simulink model "torque_control_model_2_3_2019"  (R2017b)
settings: Solver=VariableStepAuto  StartTime=0.0  StopTime=10  RelTol=1e-3
InitFcn:
  | BLDC_motor_constants_2
values from neighbouring files (symbols this model uses):
  A = [-terminal_resistance/terminal_inductance, 0, 0 ... (first row only)    [BLDC_motor_constants_2.m]    (also in forward_dynamics.m = pinv(Z) * V; inverse_dynamics.m = -pinv(Z) * v)
  B = [2/(3 * terminal_inductance), 1/(3 * terminal_inductance), 0 ... (first row only)    [BLDC_motor_constants_2.m]    (also in forward_dynamics.m = pinv(Z)/gear_ratio)
  C = [1, 0, 0 ... (first row only)    [BLDC_motor_constants_2.m]
  pole_pairs = 8    [BLDC_motor_constants_2.m]
  speed_constant = 259    [BLDC_motor_constants_2.m]
  terminal_resistance = 0.608    [BLDC_motor_constants_2.m]
  torque_constant = 36.9    [BLDC_motor_constants_2.m]
libraries: simulink x2
settings Model: Creator=Zach  LastModifiedBy=Zach

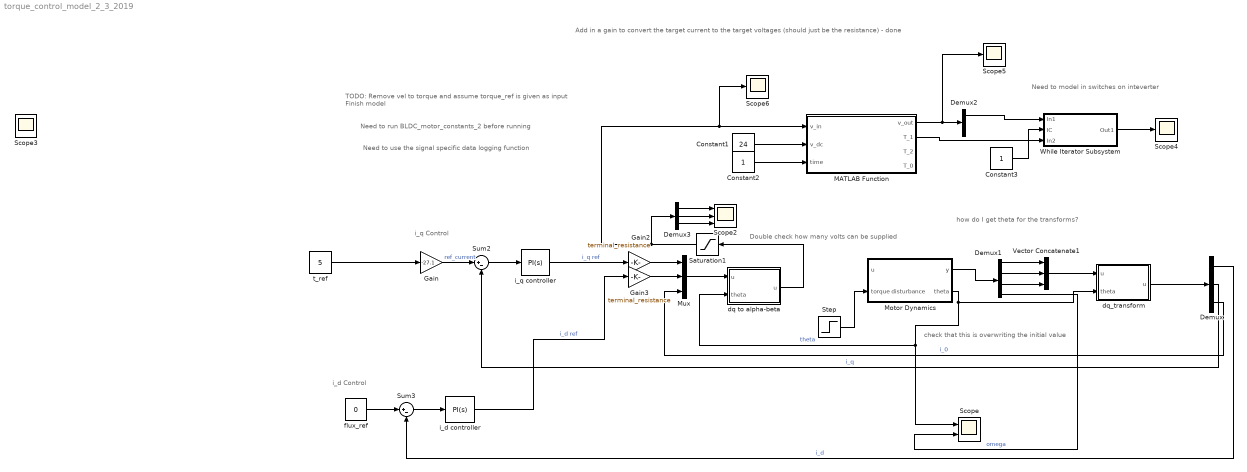
== system torque_control_model_2_3_2019 ==
  note: how do I get theta for the transforms?
  note: Need to model in switches on inteverter
  note: TODO: Remove vel to torque and assume torque_ref is given as input
      | Finish model
  note: Add in a gain to convert the target current to the target voltages (should just be the resistance) - done
  note: Need to use the signal specific data logging function
  note: check that this is overwriting the initial value
  note: i_d Control
  note: i_q Control
  note: Need to run BLDC_motor_constants_2 before running
  note: Double check how many volts can be supplied
  Constant1 : Constant  Value=24
  Constant2 : Constant
  Constant3 : Constant
  Demux : Demux  Outputs=3
  Demux1 : Demux
  Demux2 : Demux  Outputs=2
  Demux3 : Demux  Outputs=3
  Gain : Gain  Gain=-27.1
  Gain2 : Gain  Gain=terminal_resistance
  Gain3 : Gain  Gain=terminal_resistance
  MATLAB Function : MATLAB Function  TreatAsAtomicUnit=on
  Motor Dynamics : Subsystem
  Mux : Mux  Inputs=3
  Saturation1 : Saturate  UpperLimit=24  LowerLimit=-24
  Scope : Scope  NumInputPorts=2
  Scope2 : Scope  NumInputPorts=3
  Scope{3..6} (4 alike) : Scope
  Step : Step  Time=10  After=-.25  SampleTime=0
  Sum2 : Sum  Inputs=|+-
  Sum3 : Sum  Inputs=|+-
  Vector Concatenate1 : Concatenate  NumInputs=3
  While Iterator Subsystem : Subsystem  TreatAsAtomicUnit=on
  dq to alpha-beta : MATLAB Function  TreatAsAtomicUnit=on
  dq_transform : MATLAB Function  TreatAsAtomicUnit=on
  flux_ref : Constant  Value=0
  i_d controller : simulink/Continuous/PID Controller  Controller=PI  TimeDomain=Continuous-time  SampleTime=-1  IntegratorMethod=Forward Euler  FilterMethod=Forward Euler  Form=Parallel  UseFilter=on  ControllerParametersSource=internal  P=1  I=1  D=0  N=100  InitialConditionSource=internal  InitialConditionForIntegrator=0  InitialConditionForFilter=0  ExternalReset=none  LimitOutput=off  UpperSaturationLimit=inf  LowerSaturationLimit=-inf  LinearizeAsGain=on  AntiWindupMode=none  Kb=1  TrackingMode=off  Kt=1  PParamMin=[]  PParamMax=[]  IParamMin=[]  IParamMax=[]  DParamMin=[]  DParamMax=[]  NParamMin=[]  NParamMax=[]  KbParamMin=[]  KbParamMax=[]  KtParamMin=[]  KtParamMax=[]  POutMin=[]  POutMax=[]  IOutMin=[]  IOutMax=[]  DOutMin=[]  DOutMax=[]  NOutMin=[]  NOutMax=[]  KbOutMin=[]  KbOutMax=[]  KtOutMin=[]  KtOutMax=[]  IntegratorOutMin=[]  IntegratorOutMax=[]  FilterOutMin=[]  FilterOutMax=[]  SumOutMin=[]  SumOutMax=[]  SumI1OutMin=[]  SumI1OutMax=[]  SumI2OutMin=[]  SumI2OutMax=[]  SumI3OutMin=[]  SumI3OutMax=[]  SumDOutMin=[]  SumDOutMax=[]  SaturationOutMin=[]  SaturationOutMax=[]  IntegratorContinuousStateAttributes=''  IntegratorStateMustResolveToSignalObject=off  IntegratorRTWStateStorageClass=Auto  FilterContinuousStateAttributes=''  FilterStateMustResolveToSignalObject=off  FilterRTWStateStorageClass=Auto  DifferentiatorICPrevScaledInput=0  DifferentiatorOutMin=[]  DifferentiatorOutMax=[]  InitialConditionSetting=State (most efficient)  FilterDiffOutCoefMin=[]  FilterDiffOutCoefMax=[]  SumDenOutMin=[]  SumDenOutMax=[]  SumNumOutMin=[]  SumNumOutMax=[]  ReciprocalOutMin=[]  ReciprocalOutMax=[]  DivideOutMin=[]  DivideOutMax=[]  TunerSelectOption=Transfer Function Based (PID Tuner App)
  i_q controller : simulink/Continuous/PID Controller  Controller=PI  TimeDomain=Continuous-time  SampleTime=-1  IntegratorMethod=Forward Euler  FilterMethod=Forward Euler  Form=Parallel  UseFilter=on  ControllerParametersSource=internal  P=2  I=1  D=0  N=100  InitialConditionSource=internal  InitialConditionForIntegrator=0  InitialConditionForFilter=0  ExternalReset=none  LimitOutput=off  UpperSaturationLimit=inf  LowerSaturationLimit=-inf  LinearizeAsGain=on  AntiWindupMode=none  Kb=1  TrackingMode=off  Kt=1  PParamMin=[]  PParamMax=[]  IParamMin=[]  IParamMax=[]  DParamMin=[]  DParamMax=[]  NParamMin=[]  NParamMax=[]  KbParamMin=[]  KbParamMax=[]  KtParamMin=[]  KtParamMax=[]  POutMin=[]  POutMax=[]  IOutMin=[]  IOutMax=[]  DOutMin=[]  DOutMax=[]  NOutMin=[]  NOutMax=[]  KbOutMin=[]  KbOutMax=[]  KtOutMin=[]  KtOutMax=[]  IntegratorOutMin=[]  IntegratorOutMax=[]  FilterOutMin=[]  FilterOutMax=[]  SumOutMin=[]  SumOutMax=[]  SumI1OutMin=[]  SumI1OutMax=[]  SumI2OutMin=[]  SumI2OutMax=[]  SumI3OutMin=[]  SumI3OutMax=[]  SumDOutMin=[]  SumDOutMax=[]  SaturationOutMin=[]  SaturationOutMax=[]  IntegratorContinuousStateAttributes=''  IntegratorStateMustResolveToSignalObject=off  IntegratorRTWStateStorageClass=Auto  FilterContinuousStateAttributes=''  FilterStateMustResolveToSignalObject=off  FilterRTWStateStorageClass=Auto  DifferentiatorICPrevScaledInput=0  DifferentiatorOutMin=[]  DifferentiatorOutMax=[]  InitialConditionSetting=State (most efficient)  FilterDiffOutCoefMin=[]  FilterDiffOutCoefMax=[]  SumDenOutMin=[]  SumDenOutMax=[]  SumNumOutMin=[]  SumNumOutMax=[]  ReciprocalOutMin=[]  ReciprocalOutMax=[]  DivideOutMin=[]  DivideOutMax=[]  TunerSelectOption=Transfer Function Based (PID Tuner App)
  t_ref : Constant  Value=5
  wires:
  Gain/1 -> Sum2/1  "ref_current"
  Sum2/1 -> i_q controller/1
  i_q controller/1 -> Gain2/1  "i_q ref"
  Demux/2 -> Sum2/2  "i_q"
  flux_ref/1 -> Sum3/1
  Sum3/1 -> i_d controller/1
  Demux/1 -> Sum3/2  "i_d"
  i_d controller/1 -> Gain3/1  "i_d ref"
  Demux/3 -> Mux/3  "i_0"
  Step/1 -> Motor Dynamics/2(torque disturbance)
  Motor Dynamics/1(y) -> Demux1/1
  Demux1/2 -> Vector Concatenate1/2
  Demux1/1 -> Vector Concatenate1/1
  Demux1/3 -> Vector Concatenate1/3
  Motor Dynamics/2(theta) -> dq_transform/2(theta), dq to alpha-beta/2(theta), Scope/1  "theta"
  Vector Concatenate1/1 -> dq_transform/1("u ")
  dq_transform/1(u) -> Demux/1
  Demux1/4 -> Scope/2  "omega"
  Gain2/1 -> Mux/1
  Gain3/1 -> Mux/2
  Constant1/1 -> MATLAB Function/2(v_dc)
  Constant2/1 -> MATLAB Function/3(time)
  MATLAB Function/1(v_out) -> Scope5/1, Demux2/1
  Demux2/1 -> While Iterator Subsystem/1(In1)
  Constant3/1 -> While Iterator Subsystem/2(IC)
  MATLAB Function/2(T_1) -> While Iterator Subsystem/3(In2)
  Saturation1/1 -> Scope6/1, MATLAB Function/1(v_in), Demux3/1
  While Iterator Subsystem/1(Out1) -> Scope4/1
  Demux3/1 -> Scope2/1
  Demux3/2 -> Scope2/2
  Demux3/3 -> Scope2/3
  t_ref/1 -> Gain/1
  Mux/1 -> dq to alpha-beta/1("u ")
  dq to alpha-beta/1(u) -> Saturation1/1

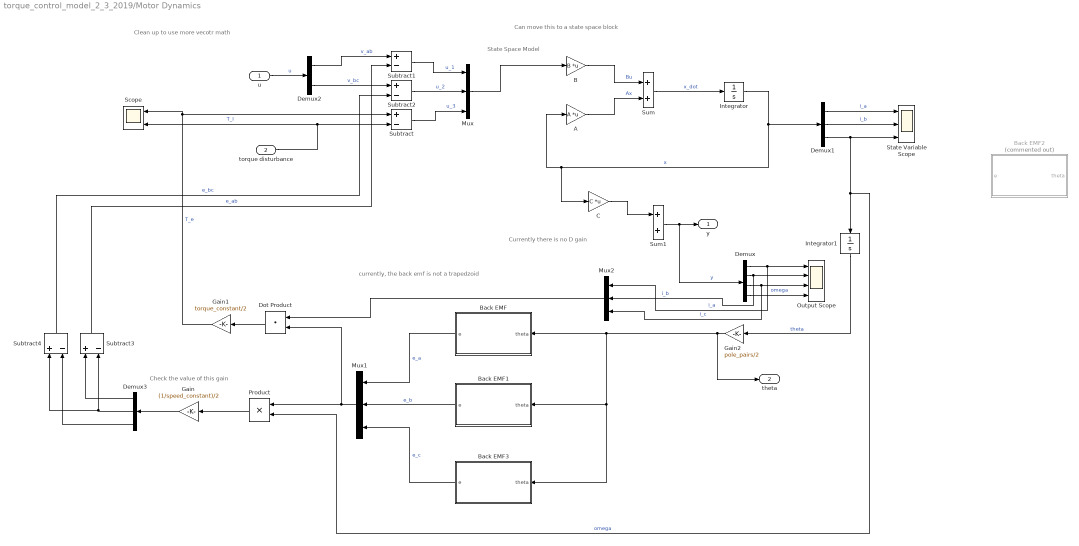
== system torque_control_model_2_3_2019/Motor Dynamics ==
  note: Check the value of this gain
  note: Can move this to a state space block
  note: Clean up to use more vecotr math
  note: currently, the back emf is not a trapedzoid
  note: Currently there is no D gain
  note: State Space Model
  u : Inport
  torque disturbance : Inport  Port=2
  A : Gain  Gain=A  Multiplication=Matrix(K*u)
  B : Gain  Gain=B  Multiplication=Matrix(K*u)
  Back EMF : Subsystem
  Back EMF1 : Subsystem
  Back EMF2 : Subsystem  Commented=on
  Back EMF3 : Subsystem
  C : Gain  Gain=C  Multiplication=Matrix(K*u)
  Demux : Demux
  Demux1 : Demux  Outputs=3
  Demux2 : Demux  Outputs=2
  Demux3 : Demux  Outputs=3
  Dot Product : DotProduct  InputSameDT=on  OutDataTypeStr=Inherit: Inherit via internal rule
  Gain : Gain  Gain=(1/speed_constant)/2
  Gain1 : Gain  Gain=torque_constant/2
  Gain2 : Gain  Gain=pole_pairs/2
  Integrator : Integrator
  Integrator1 : Integrator
  Mux : Mux  Inputs=3
  Mux1 : Mux  Inputs=3
  Mux2 : Mux  Inputs=3
  Output Scope : Scope  NumInputPorts=4
  Product : Product
  Scope : Scope  NumInputPorts=2
  State Variable Scope : Scope  NumInputPorts=3
  Subtract{,1..4} (5 alike) : Sum  Inputs=+-
  Sum : Sum
  Sum1 : Sum
  y : Outport
  theta : Outport  Port=2
  wires:
  B/1 -> Sum/1  "Bu"
  A/1 -> Sum/2  "Ax"
  Sum/1 -> Integrator/1  "x_dot"
  Integrator/1 -> Demux1/1, C/1, A/1  "x"
  C/1 -> Sum1/1
  Sum1/1 -> Demux/1, y/1  "y"
  Demux/1 -> Mux2/1, Output Scope/1  "i_a"
  Demux/2 -> Mux2/2, Output Scope/2  "i_b"
  Demux/3 -> Mux2/3, Output Scope/3  "i_c"
  Demux/4 -> Output Scope/4  "omega"
  Demux1/1 -> State Variable Scope/1  "i_a"
  Demux1/2 -> State Variable Scope/2  "i_b"
  Demux1/3 -> Product/2, Integrator1/1, State Variable Scope/3  "omega"
  Mux/1 -> B/1
  u/1 -> Demux2/1  "u"
  torque disturbance/1 -> Scope/2, Subtract/2  "T_l"
  Demux2/1 -> Subtract1/1  "v_ab"
  Demux2/2 -> Subtract2/1  "v_bc"
  Subtract2/1 -> Mux/2  "u_2"
  Subtract1/1 -> Mux/1  "u_1"
  Subtract/1 -> Mux/3  "u_3"
  Subtract3/1 -> Subtract1/2  "e_ab"
  Subtract4/1 -> Subtract2/2  "e_bc"
  Back EMF1/1(e) -> Mux1/2  "e_b"
  Back EMF/1(e) -> Mux1/1  "e_a"
  Back EMF3/1(e) -> Mux1/3  "e_c"
  Mux1/1 -> Dot Product/2, Product/1
  Product/1 -> Gain/1
  Gain/1 -> Demux3/1
  Demux3/1 -> Subtract3/1
  Demux3/2 -> Subtract4/1, Subtract3/2
  Demux3/3 -> Subtract4/2
  Mux2/1 -> Dot Product/1
  Dot Product/1 -> Gain1/1
  Gain1/1 -> Scope/1, Subtract/1  "T_e"
  Integrator1/1 -> Gain2/1  "theta"
  Gain2/1 -> theta/1, Back EMF3/1(theta), Back EMF1/1(theta), Back EMF/1(theta)

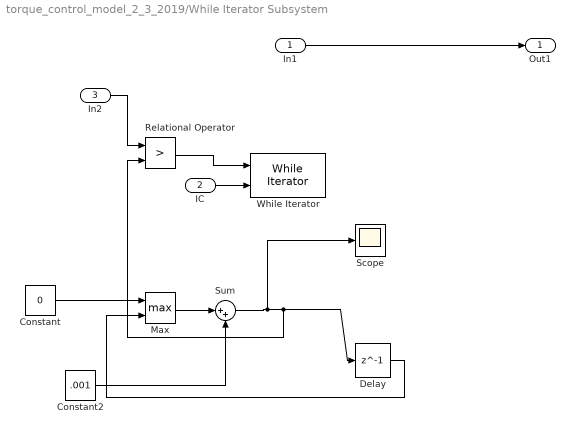
== system torque_control_model_2_3_2019/While Iterator Subsystem ==
  In1 : Inport
  IC : Inport  Port=2
  In2 : Inport  Port=3
  Constant : Constant  Value=0
  Constant2 : Constant  Value=.001
  Delay : Delay  DelayLength=1
  Max : MinMax  Function=max  Inputs=2
  Relational Operator : RelationalOperator  Operator=>  OutDataTypeStr=boolean  RndMeth=Simplest
  Scope : Scope
  Sum : Sum  Inputs=|++
  While Iterator : WhileIterator  MaxIters=-1  ResetStates=reset
  Out1 : Outport
  wires:
  IC/1 -> While Iterator/2
  In1/1 -> Out1/1
  Constant2/1 -> Sum/2
  Constant/1 -> Max/1
  Delay/1 -> Max/2
  Max/1 -> Sum/1
  Sum/1 -> Scope/1, Relational Operator/2, Delay/1
  In2/1 -> Relational Operator/1
  Relational Operator/1 -> While Iterator/1

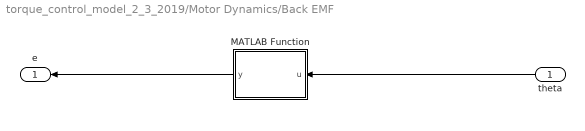
== system torque_control_model_2_3_2019/Motor Dynamics/Back EMF ==
  theta : Inport
  MATLAB Function : MATLAB Function  TreatAsAtomicUnit=on
  e : Outport
  wires:
  theta/1 -> MATLAB Function/1(u)
  MATLAB Function/1(y) -> e/1

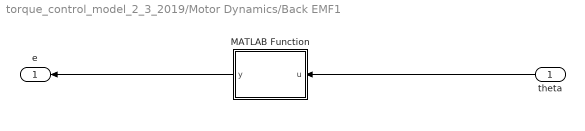
== system torque_control_model_2_3_2019/Motor Dynamics/Back EMF1 ==
  theta : Inport
  MATLAB Function : MATLAB Function  TreatAsAtomicUnit=on
  e : Outport
  wires:
  MATLAB Function/1(y) -> e/1
  theta/1 -> MATLAB Function/1(u)

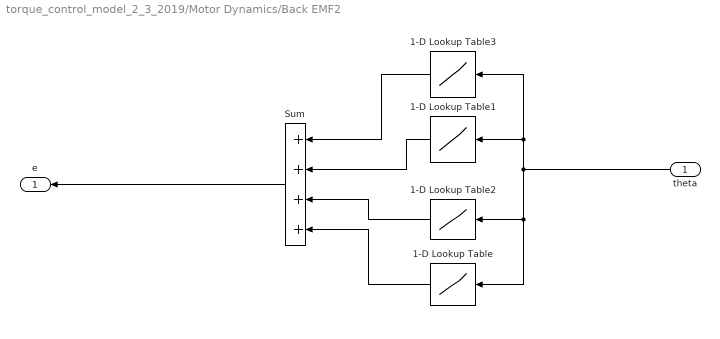
== system torque_control_model_2_3_2019/Motor Dynamics/Back EMF2 ==
  theta : Inport
  1-D Lookup Table : Lookup_n-D  NumberOfTableDimensions=1  BreakpointsForDimension1=[0, 0.000001 ,2.08, 2.09]  Table=[0, 1,1, 0]  ExtrapMethod=Clip  UseLastTableValue=on  InternalRulePriority=Speed  RndMeth=Simplest  InputSameDT=on
  1-D Lookup Table1 : Lookup_n-D  NumberOfTableDimensions=1  BreakpointsForDimension1=[3.14158, 3.1416, 5.2, 5.2333 ]  Table=[0, -1, -1, 0]  ExtrapMethod=Clip  InternalRulePriority=Speed  RndMeth=Simplest  InputSameDT=on
  1-D Lookup Table2 : Lookup_n-D  NumberOfTableDimensions=1  BreakpointsForDimension1=[2.08, 2.0943951023931953,3.14158, 3.14159]  Table=[0, 1,-0.909859317102744, 0]  ExtrapMethod=Clip  InternalRulePriority=Speed  RndMeth=Simplest  InputSameDT=on
  1-D Lookup Table3 : Lookup_n-D  NumberOfTableDimensions=1  BreakpointsForDimension1=[5.2332, 5.234, 6.27, 6.28]  Table=[0, -1,1, 0]  ExtrapMethod=Clip  InternalRulePriority=Speed  RndMeth=Simplest  InputSameDT=on
  Sum : Sum  Inputs=4
  e : Outport
  wires:
  Sum/1 -> e/1
  theta/1 -> 1-D Lookup Table1/1, 1-D Lookup Table3/1, 1-D Lookup Table2/1, 1-D Lookup Table/1
  1-D Lookup Table1/1 -> Sum/2
  1-D Lookup Table/1 -> Sum/4
  1-D Lookup Table2/1 -> Sum/3
  1-D Lookup Table3/1 -> Sum/1

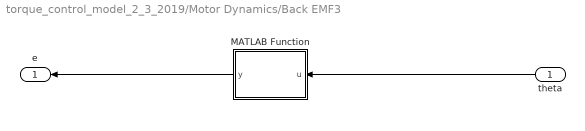
== system torque_control_model_2_3_2019/Motor Dynamics/Back EMF3 ==
  theta : Inport
  MATLAB Function : MATLAB Function  TreatAsAtomicUnit=on
  e : Outport
  wires:
  MATLAB Function/1(y) -> e/1
  theta/1 -> MATLAB Function/1(u)

== matlab function torque_control_model_2_3_2019/dq to alpha-beta ==
  data: u input; u output; theta input
function u = fcn(u, theta)
transform = ...
     [cos(theta), -sin(theta), 0;
      sin(theta), cos(theta), 0;
      0, 0, 1];
u =  transform * u;

== matlab function torque_control_model_2_3_2019/dq_transform ==
  data: u input; u output; theta input
function u = fcn(u, theta)
pole_pairs = 8; %Figure out how to pull this from the workspace
transform = sqrt(2/3) * ...
     [cos(theta * pole_pairs), cos((theta * pole_pairs) - 2*pi()/3), cos((theta * pole_pairs) + 2*pi()/3);
     -sin(theta * pole_pairs), -sin((theta * pole_pairs) - 2*pi()/3), -sin((theta * pole_pairs) + 2*pi()/3);
     1/sqrt(2), 1/sqrt(2), 1/sqrt(2)];
u = transform * u;

== matlab function torque_control_model_2_3_2019/Motor Dynamics/Back EMF/MATLAB Function ==
  data: u input; y output
function y = fcn(u)
y = 0;
u = abs(rem(u, 2*pi()));
if (0 <= u && u < 2*pi()/3)
    y = 1;
elseif (2*pi()/3 <= u && u < pi())
    y = 1 - (6/pi())*(u - (2*pi()/3)); 
elseif (pi() <= u && u < (5*pi()/3))
    y = -1;
else
    y = -1 + (6/pi())*(u - (5*pi()/3));
end

== matlab function torque_control_model_2_3_2019/Motor Dynamics/Back EMF1/MATLAB Function ==
  data: u input; y output
function y = fcn(u)
y = 0;
u = u - (2*pi()/3);
u = abs(rem(u, 2*pi()));
if (0 <= u && u < 2*pi()/3)
    y = 1;
elseif (2*pi()/3 <= u && u < pi())
    y = 1 - (6/pi())*(u - (2*pi()/3)); 
elseif (pi() <= u && u < (5*pi()/3))
    y = -1;
else
    y = -1 + (6/pi())*(u - (5*pi()/3));
end

== matlab function torque_control_model_2_3_2019/Motor Dynamics/Back EMF3/MATLAB Function ==
  data: u input; y output
function y = fcn(u)
y = 0;
u = u - (4*pi()/3);
u = abs(rem(u, 2*pi()));
if (0 <= u && u < 2*pi()/3)
    y = 1;
elseif (2*pi()/3 <= u && u < pi())
    y = 1 - (6/pi())*(u - (2*pi()/3)); 
elseif (pi() <= u && u < (5*pi()/3))
    y = -1;
else
    y = -1 + (6/pi())*(u - (5*pi()/3));
end

== matlab function torque_control_model_2_3_2019/MATLAB Function ==
  data: v_in input; v_out output; v_dc input; time input; T_1 output; T_2 output; T_0 output
function [v_out, T_1, T_2, T_0] = SVMPWM(v_in, v_dc, time)
%Time should be 1/update frequency
%Should saturate voltage input at cos(30deg)/sqrt(2) * 24
%v_in should be 3 dimensional then I apply the clark transform
%Sample every T seconds

%Input is in alpha-beta coordinate system
    x_hat = [1, 0, 0];
    v_mag = norm(v_in);
    theta = acos(dot(v_in/norm(v_in), x_hat));
    
    v_dc_r = v_mag * cos(theta);  %Make sure the units are correct
    v_dc_i = v_mag * sin(theta);  %Make sure the units are correct
    
    %% Determine which sector the vector is in
    if (theta < 60)
        sector = 1;
    elseif (theta < 120)
        sector = 2;
    elseif (theta < 180)
        sector = 3;
    elseif (theta < 240)
        sector = 4;
    elseif (theta < 300)
        sector = 5;
    else
        sector = 6;
    end
        
    %% Calculate the component strength 
    
    x_r = (v_dc * cos((60 * pi()/180) * sector));           %Real x component
    y_r = (v_dc * cos((60 * pi()/180) * (sector - 1)));     %Real y component
    
    x_i = (v_dc * sin((60* pi()/180) * sector));           %Imaginary x component
    y_i = (v_dc * sin((60* pi()/180) * (sector - 1)));     %Imaginary y component
    
    A = [x_r, y_r; x_i, y_i];
    b = A \ [v_dc_r; v_dc_i];
    v_out = (b(1) * [x_r, y_r] + b(2) * [x_i, y_i])';
    
    m = v_mag/(v_dc/2);                                        %Modulation Index
    
    T_1 = (sqrt(3)/2) * m * time * sin(pi()/3 - theta);        %Time for active vector 1
    T_2 = (sqrt(3)/2) * m * time * sin(theta);                 %Time for active vector 2
    T_0 = time - (T_1 + T_2)/2;                                %Time for zero vector
    
    %% Generate switiching times for each switch
    switch sector
        case 1
            s_1 = T_1 + T_2 + T_0/2;
            s_3 = T_2 + T_0/2;
            s_5 = T_0/2;
            
            s_4 = T_0/2;
            s_6 = T_1 + T_0/2;
            s_2 = T_1 + T_2 + T_0/2;
        case 2
        case 3
        case 4
        case 5
        case 5
        case 6
    end
    
end
    
%% Refrences:
%https://hvdc.ca/webhelp/Master_Library_Models/HVDC_and_FACTS/Space_Vector_Modulation/SVM_Theory.htm
%https://www.switchcraft.org/learning/2017/3/15/space-vector-pwm-intro
%lecture 25 ohio state PWM svm ppt
